simulink model "ISEmizgenj1sat"  (R2015a)
settings: Solver=ode45  StartTime=0.0  StopTime=10.0  RelTol=1e-3
values from neighbouring files (symbols this model uses):
  Kimiz2 = x(2)    [genetic.m]
  Kpmiz2 = x(1)    [genetic.m]
settings Model: Creator=PC  LastModifiedBy=PC

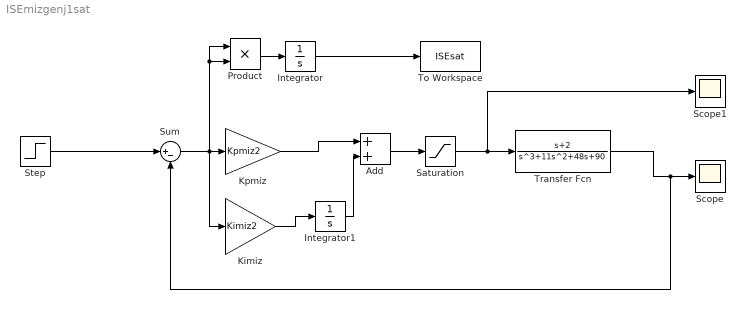
== system ISEmizgenj1sat ==
  Add : Sum
  Integrator : Integrator
  Integrator1 : Integrator
  Kimiz : Gain  Gain=Kimiz2
  Kpmiz : Gain  Gain=Kpmiz2
  Product : Product
  Saturation : Saturate  UpperLimit=90  LowerLimit=0
  Scope : Scope
  Scope1 : Scope
  Step : Step  SampleTime=0
  Sum : Sum  Inputs=|+-
  To Workspace : ToWorkspace  VariableName=ISEsat  SampleTime=-1
  Transfer Fcn : TransferFcn  Numerator=[1 2]  Denominator=[1 11 48 90]
  wires:
  Sum/1 -> Product/2, Product/1, Kpmiz/1, Kimiz/1
  Step/1 -> Sum/1
  Product/1 -> Integrator/1
  Integrator/1 -> To Workspace/1
  Kimiz/1 -> Integrator1/1
  Integrator1/1 -> Add/2
  Kpmiz/1 -> Add/1
  Add/1 -> Saturation/1
  Transfer Fcn/1 -> Sum/2, Scope/1
  Saturation/1 -> Scope1/1, Transfer Fcn/1
